simulink model "Subsystem"  (R2020b)
settings: Solver=VariableStepAuto  StartTime=0.0  StopTime=10.0  RelTol=1e-3
settings Model: Creator=HP  LastModifiedBy=HP
settings DataIOCC: SaveOutput=off  SaveTime=off

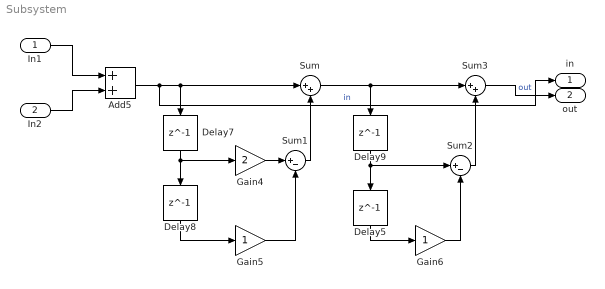
== system Subsystem ==
  In1 : Inport  OutDataTypeStr=double  PortDimensions=1  SampleTime=0
  In2 : Inport  Port=2  OutDataTypeStr=double  PortDimensions=1  SampleTime=0
  Add5 : Sum
  Delay{5,7..9} (4 alike) : Delay  DelayLength=1
  Gain4 : Gain  Gain=2
  Gain5 : Gain
  Gain6 : Gain
  Sum : Sum  Inputs=|++
  Sum1 : Sum  Inputs=|+-
  Sum2 : Sum  Inputs=|+-
  Sum3 : Sum  Inputs=|++
  in : Outport  OutDataTypeStr=double  PortDimensions=1  SampleTime=0
  out : Outport  Port=2  OutDataTypeStr=double  PortDimensions=1  SampleTime=0
  wires:
  Delay9/1 -> Delay5/1, Sum2/1
  Sum2/1 -> Sum3/2
  Add5/1 -> Sum/1, Delay7/1, in/1  "in"
  Gain4/1 -> Sum1/1
  Sum/1 -> Sum3/1, Delay9/1
  Delay8/1 -> Gain5/1
  Gain5/1 -> Sum1/2
  Gain6/1 -> Sum2/2
  Delay5/1 -> Gain6/1
  Sum1/1 -> Sum/2
  Delay7/1 -> Gain4/1, Delay8/1
  In1/1 -> Add5/1
  Sum3/1 -> out/1  "out"
  In2/1 -> Add5/2
